simulink model "Car_Lighting_ControlSystem"  (R2023b)
settings: Solver=FixedStepDiscrete  StartTime=0.0  StopTime=inf  FixedStep=10e-3  RelTol=1e-3  EnableMultiTasking=on
libraries: arduinolib x5
settings Model: ExtModeTrigDuration=2  Creator=reemb  LastModifiedBy=reemb
settings OptimizationCC: EnhancedBackFolding=on  PassReuseOutputArgsAs=Individual arguments  ZeroExternalMemoryAtStartup=off  ZeroInternalMemoryAtStartup=off  MaxStackSize=64  OptimizeBlockOrder=speed  DifferentSizesBufferReuse=on  OptimizationCustomize=off  EfficientTunableParamExpr=on
settings DebuggingCC: ParameterTunabilityLossMsg=error
settings HardwareCC: ProdBitPerInt=16  ProdBitPerPointer=16  ProdBitPerSizeT=16  ProdBitPerPtrDiffT=16  ProdLargestAtomicFloat=None  ProdWordSize=8  ProdHWDeviceType=Atmel->AVR
settings SFSimCC: MATLABDynamicMemAlloc=off
settings RTWCC: Description=Embedded Coder  SystemTargetFile=ert.tlc  HardwareBoard=Arduino Uno  TemplateMakefile=ert_default_tmf  Toolchain=Arduino AVR  BuildConfiguration=Faster Runs
settings CodeAppCC: ForceParamTrailComments=on  IgnoreCustomStorageClasses=off  OperatorAnnotations=on  SimulinkDataObjDesc=on  SFDataObjDesc=on  InsertBlockDesc=on
settings ERTTargetCC: SupportContinuousTime=on  SupportVariableSizeSignals=on  ExtModeTransport=3  ExtModeStaticAlloc=on  ExtModeAutomaticAllocSize=off  ExtModeStaticAllocSize=250  ExtModeMexFile=ext_xcp  ExtModeIntrfLevel=Level2 - Open

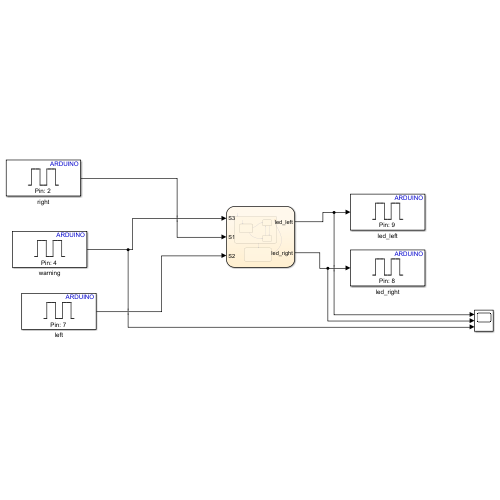
[thumbnail: Simulink's stored preview of the top-level diagram]
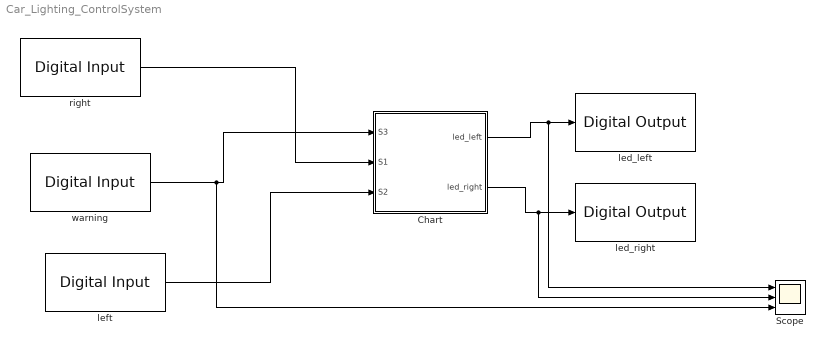
== system Car_Lighting_ControlSystem ==
  Chart : Stateflow chart  TreatAsAtomicUnit=on
  Scope : Scope  NumInputPorts=3
  led_left : arduinolib/Digital Output  pinNumber=9  Direction=output  blockPlatform=arduino
  led_right : arduinolib/Digital Output  pinNumber=8  Direction=output  blockPlatform=arduino
  left : arduinolib/Digital Input  pinNumber=7  mode=Input Pullup  Direction=input  SampleTime=0.1  blockPlatform=arduino
  right : arduinolib/Digital Input  pinNumber=2  mode=Input Pullup  Direction=input  SampleTime=0.1  blockPlatform=arduino
  warning : arduinolib/Digital Input  pinNumber=4  mode=Input Pullup  Direction=input  SampleTime=0.1  blockPlatform=arduino
  wires:
  warning/1 -> Scope/3, Chart/1(S3)
  right/1 -> Chart/2(S1)
  left/1 -> Chart/3(S2)
  Chart/1(led_left) -> Scope/1, led_left/1
  Chart/2(led_right) -> Scope/2, led_right/1

== stateflow chart Car_Lighting_ControlSystem/Chart ==
  state NORMAL
    state RIGHT
      entry:
      led_right = 1;
      led_left = 0;
    state IDEAL
      entry: led_right = 0;
      led_left = 0;
    state LEFT
      entry:
      led_left = 1;
      led_right = 0;
    (default) -> IDEAL
    IDEAL -> RIGHT [order 1] : [S1 == 0]
    LEFT -> RIGHT : [S1 == 0]
    RIGHT -> LEFT : [S2 == 0]
    IDEAL -> LEFT [order 2] : [S2 == 0]
  state WARNING
    entry:
    led_right = 1;
    led_left = 1;
  (default) -> NORMAL
  WARNING -> (history) : [S3 == 0]
  NORMAL -> WARNING : [S3 == 0]
  data: led_left output; led_right output; S3 input; S1 input; S2 input
